simulink model "ThesisSimulink"  (R2022b)
settings: Solver=VariableStepAuto  StartTime=0.0  StopTime=1  RelTol=1e-3
settings Model: Creator=ranafaheemiftikhar  LastModifiedBy=ranafaheemiftikhar

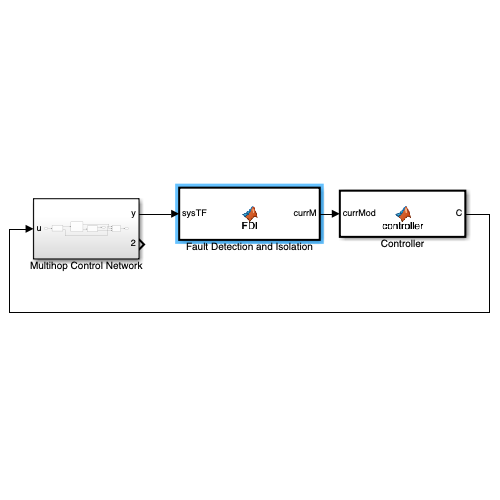
[thumbnail: Simulink's stored preview of the top-level diagram]
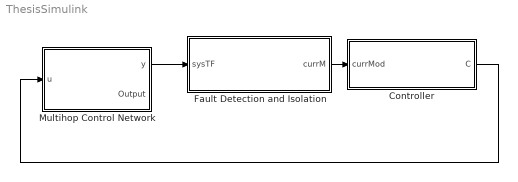
== system ThesisSimulink ==
  Controller : MATLAB Function  TreatAsAtomicUnit=on
  Fault Detection and Isolation : MATLAB Function  TreatAsAtomicUnit=on
  Multihop Control Network : Subsystem
  wires:
  Multihop Control Network/1(y) -> Fault Detection and Isolation/1(sysTF)
  Fault Detection and Isolation/1(currM) -> Controller/1(currMod)
  Controller/1(C) -> Multihop Control Network/1(u)

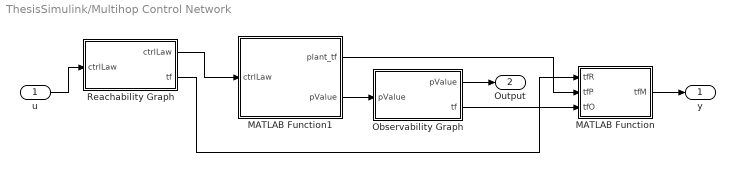
== system ThesisSimulink/Multihop Control Network ==
  u : Inport
  MATLAB Function : MATLAB Function  TreatAsAtomicUnit=on
  MATLAB Function1 : MATLAB Function  TreatAsAtomicUnit=on
  Observability Graph : MATLAB Function  TreatAsAtomicUnit=on
  Reachability Graph : MATLAB Function  TreatAsAtomicUnit=on
  y : Outport
  Output : Outport  Port=2
  wires:
  u/1 -> Reachability Graph/1("ctrlLaw ")
  Reachability Graph/1(ctrlLaw) -> MATLAB Function1/1(ctrlLaw)
  MATLAB Function1/2(pValue) -> Observability Graph/1("pValue ")
  MATLAB Function1/1(plant_tf) -> MATLAB Function/2(tfP)
  Reachability Graph/2(tf) -> MATLAB Function/1(tfR)
  Observability Graph/2(tf) -> MATLAB Function/3(tfO)
  Observability Graph/1(pValue) -> Output/1
  MATLAB Function/1(tfM) -> y/1

== matlab function ThesisSimulink/Multihop Control Network/Reachability Graph ==
  data: ctrlLaw output; tf output; ctrlLaw input
function [ctrlLaw,tf] = Gr_Tf(ctrlLaw)
s = [1,1,1,2,3,4];
d = [2,3,4,5,5,5];
sched_func = {[1,2],[1,3],[1,4],[2,5],[3,5],[4,5]};
[paths,G] = createGraph(s,d,50);
[tf_empty,transfer_function] = transferFunctionCalculate(paths, sched_func,G);

if tf_empty
    ctrlLaw = 0;
    tf = 0; 
else
    tf = transfer_function;
end

== matlab function ThesisSimulink/Fault Detection and Isolation ==
  data: sysTF input; currM output
function currM = FDI(sysTF)
disp(sysTF)
currM = sysTF;

== matlab function ThesisSimulink/Controller ==
  data: currMod input; C output
function C = controller(currMod)

C = currMod;

== matlab function ThesisSimulink/Multihop Control Network/MATLAB Function ==
  data: tfR input; tfM output; tfP input; tfO input
function tfM = systemTF(tfR, tfP, tfO)
    tfM = tfR*tfP*tfO;

== matlab function ThesisSimulink/Multihop Control Network/MATLAB Function1 ==
  data: ctrlLaw input; plant_tf output; pValue output
function [plant_tf,pValue] = plant(ctrlLaw)
    num_p = 0.5;
    den_p = [1, -0.8];
    plant_tf = tf(num_p, den_p, 1, 'variable', 'z'); 
    pValue = num_p;

== matlab function ThesisSimulink/Multihop Control Network/Observability Graph ==
  data: pValue output; pValue input; tf output
function [pValue,tf] = Go_Tf(pValue)

s = [1,1,1,2,3,4];
d = [2,3,4,5,5,5];
sched_func = {[1,2],[1,3],[1,4],[2,5],[3,5],[4,5]};
[paths,G] = createGraph(s,d,50);
[tf_empty,transfer_function] = transferFunctionCalculate(paths, sched_func,G);

if tf_empty
    pValue = 0;
    tf = 0; 
else
    tf = transfer_function;
end
